simulink model "BalloonDrift"  (R2020a)
settings: Solver=VariableStepAuto  StartTime=0.0  StopTime=1800  FixedStep=0.4  RelTol=1e-3
undefined symbols (not defined in the file or in its folder): HDBK, MIL
libraries: aerolibatmos2 x1, simulink x1
settings Model: Creator=j90xb  LastModifiedBy=jasch

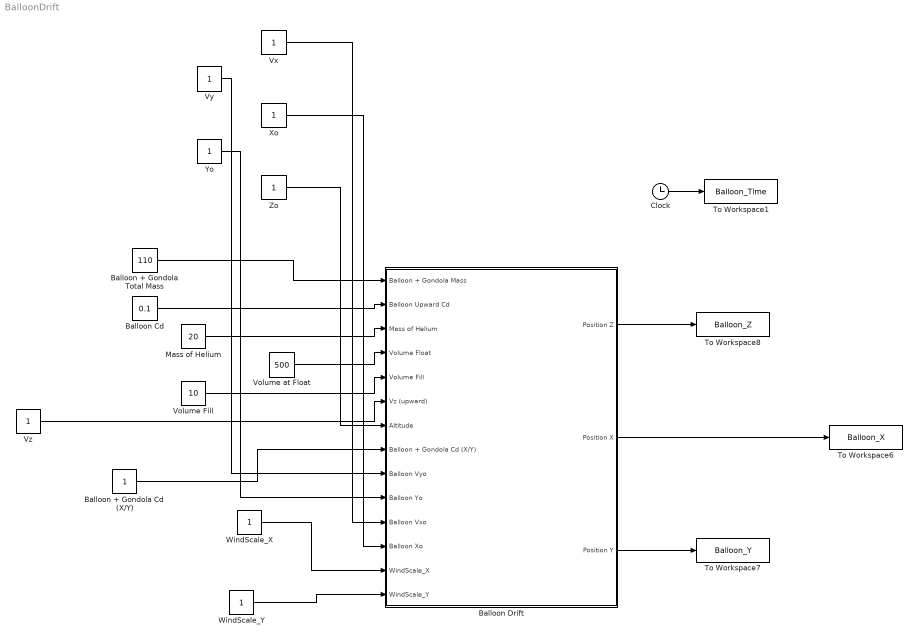
== system BalloonDrift ==
  Balloon + Gondola Cd (X/Y) : Constant
  Balloon + Gondola Total Mass : Constant  Value=110
  Balloon Cd : Constant  Value=0.1
  Balloon Drift : Subsystem  TreatAsAtomicUnit=on
  Clock : Clock
  Mass of Helium : Constant  Value=20
  To Workspace1 : ToWorkspace  VariableName=Balloon_Time  SampleTime=-1
  To Workspace6 : ToWorkspace  VariableName=Balloon_X  SampleTime=-1
  To Workspace7 : ToWorkspace  VariableName=Balloon_Y  SampleTime=-1
  To Workspace8 : ToWorkspace  VariableName=Balloon_Z  SampleTime=-1
  Volume Fill : Constant  Value=10
  Volume at Float : Constant  Value=500
  Vx : Constant
  Vy : Constant
  Vz : Constant
  WindScale_X : Constant
  WindScale_Y : Constant
  Xo : Constant
  Yo : Constant
  Zo : Constant
  wires:
  Vx/1 -> Balloon Drift/11(Balloon Vxo)
  Yo/1 -> Balloon Drift/10(Balloon Yo)
  Vy/1 -> Balloon Drift/9(Balloon Vyo)
  Zo/1 -> Balloon Drift/7(Altitude)
  Xo/1 -> Balloon Drift/12(Balloon Xo)
  Balloon Drift/2(Position X) -> To Workspace6/1
  Balloon Drift/1(Position Z) -> To Workspace8/1
  Balloon Drift/3(Position Y) -> To Workspace7/1
  Vz/1 -> Balloon Drift/6(Vz (upward))
  Balloon + Gondola Cd (X/Y)/1 -> Balloon Drift/8(Balloon + Gondola Cd (X/Y))
  Balloon + Gondola Total Mass/1 -> Balloon Drift/1(Balloon + Gondola Mass)
  Balloon Cd/1 -> Balloon Drift/2(Balloon Upward Cd)
  Mass of Helium/1 -> Balloon Drift/3(Mass of Helium)
  Volume at Float/1 -> Balloon Drift/4(Volume Float)
  Volume Fill/1 -> Balloon Drift/5(Volume Fill)
  Clock/1 -> To Workspace1/1
  WindScale_X/1 -> Balloon Drift/13(WindScale_X)
  WindScale_Y/1 -> Balloon Drift/14(WindScale_Y)

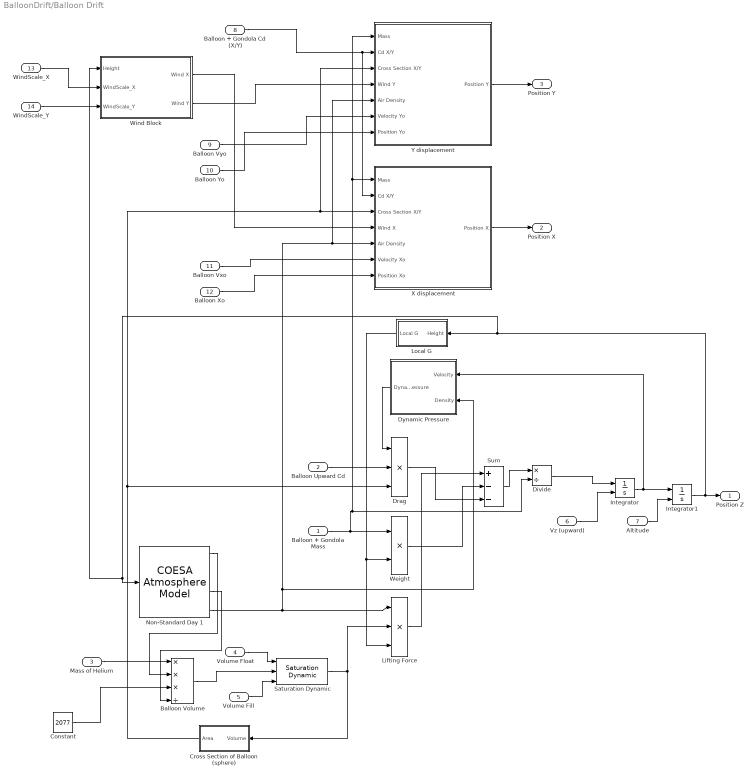
== system BalloonDrift/Balloon Drift ==
  Balloon + Gondola Mass : Inport
  Balloon Upward Cd : Inport  Port=2
  Mass of Helium : Inport  Port=3
  Volume Float : Inport  Port=4
  Volume Fill : Inport  Port=5
  Vz (upward) : Inport  Port=6
  Altitude : Inport  Port=7
  Balloon + Gondola Cd (X/Y) : Inport  Port=8
  Balloon Vyo : Inport  Port=9
  Balloon Yo : Inport  Port=10
  Balloon Vxo : Inport  Port=11
  Balloon Xo : Inport  Port=12
  WindScale_X : Inport  Port=13
  WindScale_Y : Inport  Port=14
  Balloon Volume : Product  Inputs=***/
  Constant : Constant  Value=2077
  Cross Section of Balloon (sphere) : Subsystem
  Divide : Product  Inputs=*/
  Drag : Product  Inputs=3
  Dynamic Pressure : Subsystem  TreatAsAtomicUnit=on
  Integrator : Integrator  InitialConditionSource=external
  Integrator1 : Integrator  InitialConditionSource=external
  Lifting Force : Product  Inputs=3
  Local G : Subsystem
  Non-Standard Day 1 : aerolibatmos2/COESA Atmosphere Model  units=Metric (MKS)  spec=MIL-HDBK-310  model=Profile  profile_var=High temperature  profile_percent=1%  profile_alt=5 km (16404 ft)  envelope_var=High temperature  envelope_percent=1%  action=Warning
  Saturation Dynamic : simulink/Discontinuities/Saturation Dynamic  OutMin=[]  OutMax=[]  OutDataTypeStr=Inherit: Same as second input  OutDataType=fixdt(1, 16)  OutScaling=2^-10  DoSatur=off
  Sum : Sum  Inputs=+--
  Weight : Product
  Wind Block : Subsystem  TreatAsAtomicUnit=on
  X displacement : Subsystem  TreatAsAtomicUnit=on
  Y displacement : Subsystem  TreatAsAtomicUnit=on
  Position Z : Outport
  Position X : Outport  Port=2
  Position Y : Outport  Port=3
  wires:
  Sum/1 -> Divide/1
  Local G/1(Local G) -> Weight/2, Lifting Force/3
  Balloon + Gondola Mass/1 -> X displacement/1(Mass), Y displacement/1(Mass), Divide/2, Weight/1
  Weight/1 -> Sum/2
  Dynamic Pressure/1(Dynamic Pressure) -> Drag/1
  Balloon Upward Cd/1 -> Drag/2
  Drag/1 -> Sum/3
  Lifting Force/1 -> Sum/1
  Mass of Helium/1 -> Balloon Volume/1
  Non-Standard Day 1/1 -> Balloon Volume/2
  Balloon Volume/1 -> Saturation Dynamic/2
  Saturation Dynamic/1 -> Cross Section of Balloon (sphere)/1(Volume), Lifting Force/2
  Volume Float/1 -> Saturation Dynamic/1
  Volume Fill/1 -> Saturation Dynamic/3
  Integrator/1 -> Dynamic Pressure/1("Velocity "), Integrator1/1
  Vz (upward)/1 -> Integrator/2
  Altitude/1 -> Integrator1/2
  Integrator1/1 -> Non-Standard Day 1/1, Wind Block/1(Height), Local G/1(Height), Position Z/1
  Divide/1 -> Integrator/1
  X displacement/1(Position X) -> Position X/1
  Y displacement/1(Position Y) -> Position Y/1
  Cross Section of Balloon (sphere)/1(Area) -> Drag/3, Y displacement/3(Cross Section X/Y), X displacement/3(Cross Section X/Y)
  Non-Standard Day 1/4 -> Y displacement/5(Air Density), X displacement/5(Air Density), Dynamic Pressure/2(Density), Lifting Force/1
  Balloon + Gondola Cd (X/Y)/1 -> X displacement/2(Cd X/Y), Y displacement/2(Cd X/Y)
  Balloon Vyo/1 -> Y displacement/6(Velocity Yo)
  Balloon Yo/1 -> Y displacement/7(Position Yo)
  Balloon Vxo/1 -> X displacement/6(Velocity Xo)
  Balloon Xo/1 -> X displacement/7(Position Xo)
  Non-Standard Day 1/3 -> Balloon Volume/4
  Constant/1 -> Balloon Volume/3
  Wind Block/1(Wind X) -> X displacement/4(Wind X)
  Wind Block/2(Wind Y) -> Y displacement/4(Wind Y)
  WindScale_X/1 -> Wind Block/2(WindScale_X)
  WindScale_Y/1 -> Wind Block/3(WindScale_Y)

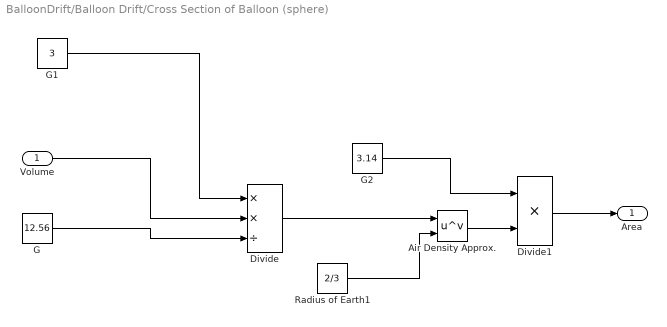
== system BalloonDrift/Balloon Drift/Cross Section of Balloon (sphere) ==
  Volume : Inport
  Air Density Approx. : Math  Operator=pow  OutMin=0  OutMax=10000  SaturateOnIntegerOverflow=on
  Divide : Product  Inputs=**/
  Divide1 : Product  Inputs=**
  G : Constant  Value=12.56
  G1 : Constant  Value=3
  G2 : Constant  Value=3.14
  Radius of Earth1 : Constant  Value=2/3
  Area : Outport  VectorParamsAs1DForOutWhenUnconnected=off
  wires:
  Volume/1 -> Divide/2
  Divide/1 -> Air Density Approx./1
  Radius of Earth1/1 -> Air Density Approx./2
  G/1 -> Divide/3
  G1/1 -> Divide/1
  Air Density Approx./1 -> Divide1/2
  Divide1/1 -> Area/1
  G2/1 -> Divide1/1

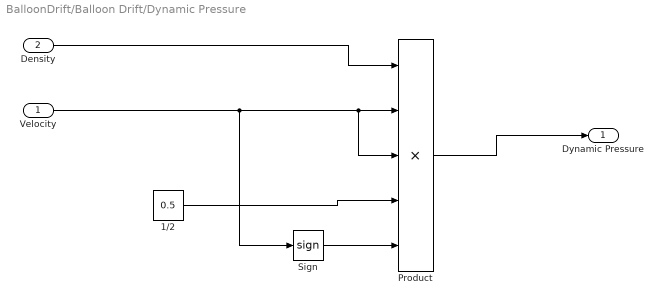
== system BalloonDrift/Balloon Drift/Dynamic Pressure ==
  "Velocity " : Inport
  Density : Inport  Port=2
  1/2 : Constant  Value=0.5
  Product : Product  Inputs=5
  Sign : Signum
  Dynamic Pressure : Outport
  wires:
  "Velocity "/1 -> Sign/1, Product/2, Product/3
  Density/1 -> Product/1
  Product/1 -> Dynamic Pressure/1
  1/2/1 -> Product/4
  Sign/1 -> Product/5

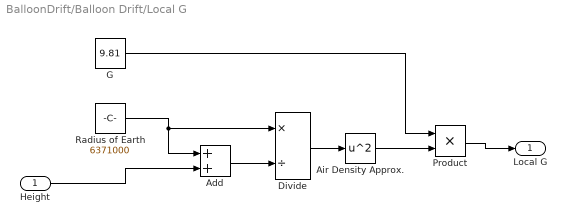
== system BalloonDrift/Balloon Drift/Local G ==
  Height : Inport
  Add : Sum
  Air Density Approx. : Math  Operator=square  SignedPower=on  OutMin=0  OutMax=10000  SaturateOnIntegerOverflow=on
  Divide : Product  Inputs=*/
  G : Constant  Value=9.81
  Product : Product
  Radius of Earth : Constant  Value=6371000
  Local G : Outport  VectorParamsAs1DForOutWhenUnconnected=off
  wires:
  Radius of Earth/1 -> Divide/1, Add/1
  Height/1 -> Add/2
  Add/1 -> Divide/2
  Divide/1 -> Air Density Approx./1
  Air Density Approx./1 -> Product/2
  Product/1 -> Local G/1
  G/1 -> Product/1

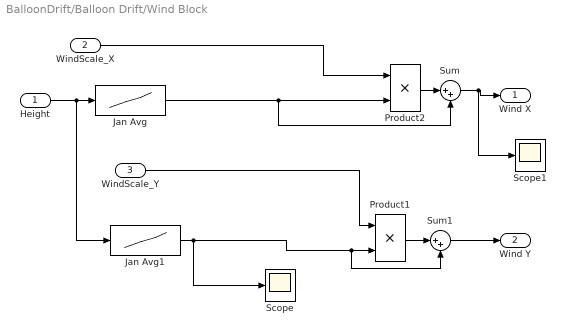
== system BalloonDrift/Balloon Drift/Wind Block ==
  Height : Inport
  WindScale_X : Inport  Port=2
  WindScale_Y : Inport  Port=3
  Jan Avg : Lookup_n-D  NumberOfTableDimensions=1  BreakpointsForDimension1=[0,5000,10000,15000,20000,24000,100000]  IndexSearchMethod=Linear search  Table=[2,17,30,22,5,2,0]  InterpMethod=Cubic spline  ExtrapMethod=Clip  UseLastTableValue=on  InternalRulePriority=Speed  RndMeth=Simplest  InputSameDT=on
  Jan Avg1 : Lookup_n-D  NumberOfTableDimensions=1  BreakpointsForDimension1=[0,5000,10000,15000,20000,24000,100000]  Table=[2,17,30,22,5,2,0]  InterpMethod=Cubic spline  ExtrapMethod=Clip  UseLastTableValue=on  InternalRulePriority=Speed  RndMeth=Simplest  InputSameDT=on
  Product1 : Product
  Product2 : Product
  Scope : Scope
  Scope1 : Scope
  Sum : Sum  Inputs=|++
  Sum1 : Sum  Inputs=|++
  Wind X : Outport
  Wind Y : Outport  Port=2
  wires:
  Height/1 -> Jan Avg1/1, Jan Avg/1
  Jan Avg/1 -> Sum/2, Product2/2
  Jan Avg1/1 -> Scope/1, Sum1/2, Product1/2
  WindScale_X/1 -> Product2/1
  WindScale_Y/1 -> Product1/1
  Product2/1 -> Sum/1
  Sum/1 -> Scope1/1, Wind X/1
  Product1/1 -> Sum1/1
  Sum1/1 -> Wind Y/1

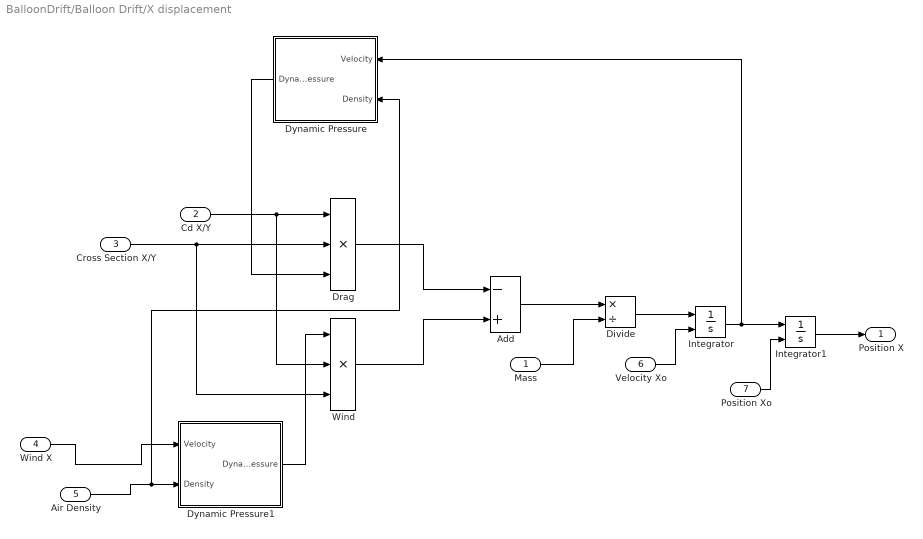
== system BalloonDrift/Balloon Drift/X displacement ==
  Mass : Inport
  Cd X/Y : Inport  Port=2
  Cross Section X/Y : Inport  Port=3
  Wind X : Inport  Port=4
  Air Density : Inport  Port=5
  Velocity Xo : Inport  Port=6
  Position Xo : Inport  Port=7
  Add : Sum  Inputs=-+
  Divide : Product  Inputs=*/
  Drag : Product  Inputs=3
  Dynamic Pressure : Subsystem  TreatAsAtomicUnit=on
  Dynamic Pressure1 : Subsystem  TreatAsAtomicUnit=on
  Integrator : Integrator  InitialConditionSource=external
  Integrator1 : Integrator  InitialConditionSource=external
  Wind : Product  Inputs=3
  Position X : Outport
  wires:
  Add/1 -> Divide/1
  Mass/1 -> Divide/2
  Wind/1 -> Add/2
  Drag/1 -> Add/1
  Cd X/Y/1 -> Wind/2, Drag/1
  Cross Section X/Y/1 -> Wind/3, Drag/2
  Dynamic Pressure/1(Dynamic Pressure) -> Drag/3
  Divide/1 -> Integrator/1
  Integrator/1 -> Dynamic Pressure/1("Velocity "), Integrator1/1
  Integrator1/1 -> Position X/1
  Dynamic Pressure1/1(Dynamic Pressure) -> Wind/1
  Air Density/1 -> Dynamic Pressure/2(Density), Dynamic Pressure1/2(Density)
  Velocity Xo/1 -> Integrator/2
  Position Xo/1 -> Integrator1/2
  Wind X/1 -> Dynamic Pressure1/1("Velocity ")

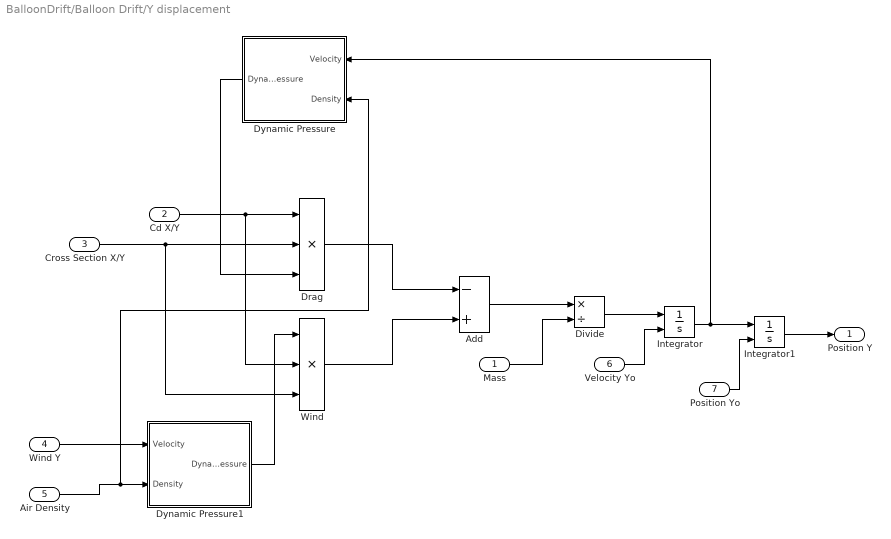
== system BalloonDrift/Balloon Drift/Y displacement ==
  Mass : Inport
  Cd X/Y : Inport  Port=2
  Cross Section X/Y : Inport  Port=3
  Wind Y : Inport  Port=4
  Air Density : Inport  Port=5
  Velocity Yo : Inport  Port=6
  Position Yo : Inport  Port=7
  Add : Sum  Inputs=-+
  Divide : Product  Inputs=*/
  Drag : Product  Inputs=3
  Dynamic Pressure : Subsystem  TreatAsAtomicUnit=on
  Dynamic Pressure1 : Subsystem  TreatAsAtomicUnit=on
  Integrator : Integrator  InitialConditionSource=external
  Integrator1 : Integrator  InitialConditionSource=external
  Wind : Product  Inputs=3
  Position Y : Outport
  wires:
  Add/1 -> Divide/1
  Mass/1 -> Divide/2
  Wind/1 -> Add/2
  Drag/1 -> Add/1
  Cd X/Y/1 -> Wind/2, Drag/1
  Cross Section X/Y/1 -> Wind/3, Drag/2
  Dynamic Pressure/1(Dynamic Pressure) -> Drag/3
  Divide/1 -> Integrator/1
  Integrator/1 -> Dynamic Pressure/1("Velocity "), Integrator1/1
  Integrator1/1 -> Position Y/1
  Dynamic Pressure1/1(Dynamic Pressure) -> Wind/1
  Wind Y/1 -> Dynamic Pressure1/1("Velocity ")
  Air Density/1 -> Dynamic Pressure/2(Density), Dynamic Pressure1/2(Density)
  Velocity Yo/1 -> Integrator/2
  Position Yo/1 -> Integrator1/2

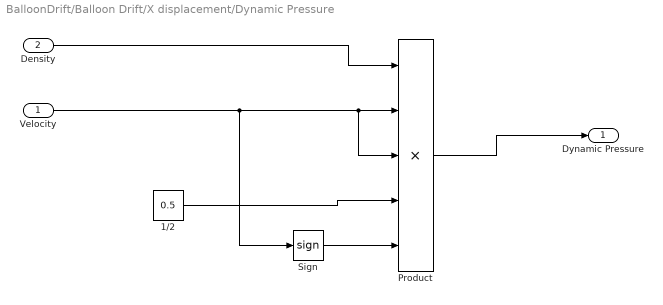
== system BalloonDrift/Balloon Drift/X displacement/Dynamic Pressure ==
  "Velocity " : Inport
  Density : Inport  Port=2
  1/2 : Constant  Value=0.5
  Product : Product  Inputs=5
  Sign : Signum
  Dynamic Pressure : Outport
  wires:
  "Velocity "/1 -> Sign/1, Product/2, Product/3
  Density/1 -> Product/1
  Product/1 -> Dynamic Pressure/1
  1/2/1 -> Product/4
  Sign/1 -> Product/5

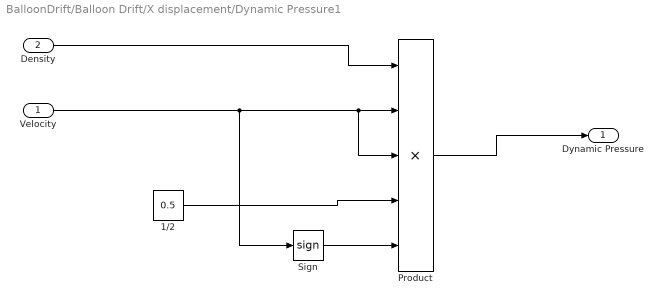
== system BalloonDrift/Balloon Drift/X displacement/Dynamic Pressure1 ==
  "Velocity " : Inport
  Density : Inport  Port=2
  1/2 : Constant  Value=0.5
  Product : Product  Inputs=5
  Sign : Signum
  Dynamic Pressure : Outport
  wires:
  "Velocity "/1 -> Sign/1, Product/2, Product/3
  Density/1 -> Product/1
  Product/1 -> Dynamic Pressure/1
  1/2/1 -> Product/4
  Sign/1 -> Product/5

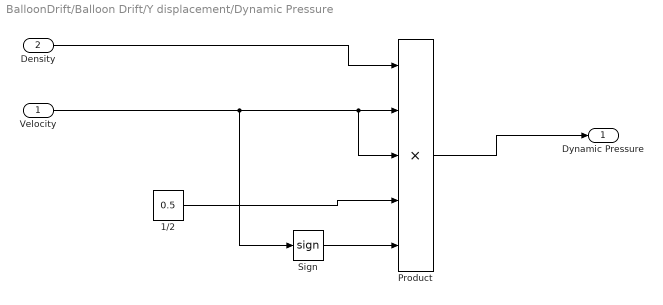
== system BalloonDrift/Balloon Drift/Y displacement/Dynamic Pressure ==
  "Velocity " : Inport
  Density : Inport  Port=2
  1/2 : Constant  Value=0.5
  Product : Product  Inputs=5
  Sign : Signum
  Dynamic Pressure : Outport
  wires:
  "Velocity "/1 -> Sign/1, Product/2, Product/3
  Density/1 -> Product/1
  Product/1 -> Dynamic Pressure/1
  1/2/1 -> Product/4
  Sign/1 -> Product/5

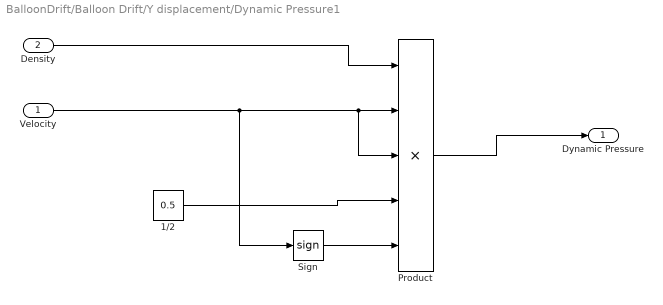
== system BalloonDrift/Balloon Drift/Y displacement/Dynamic Pressure1 ==
  "Velocity " : Inport
  Density : Inport  Port=2
  1/2 : Constant  Value=0.5
  Product : Product  Inputs=5
  Sign : Signum
  Dynamic Pressure : Outport
  wires:
  "Velocity "/1 -> Sign/1, Product/2, Product/3
  Density/1 -> Product/1
  Product/1 -> Dynamic Pressure/1
  1/2/1 -> Product/4
  Sign/1 -> Product/5
